simulink model "twoDofSmc"  (R2023b)
settings: Solver=VariableStepAuto  StartTime=0.0  StopTime=10.0  RelTol=1e-3
settings Model: Creator=Egraweb  LastModifiedBy=Egraweb
settings DebuggingCC: UnderSpecifiedDimensionMsg=warning

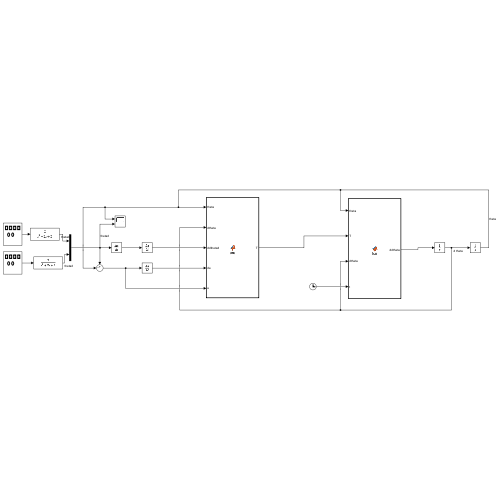
[thumbnail: Simulink's stored preview of the top-level diagram]
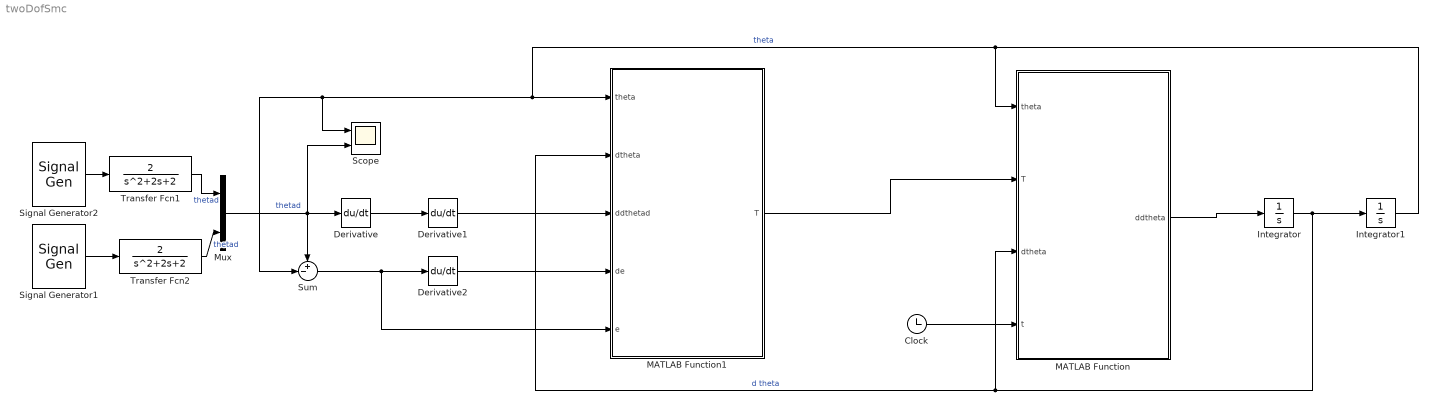
== system twoDofSmc ==
  Clock : Clock
  Derivative : Derivative
  Derivative1 : Derivative
  Derivative2 : Derivative
  Integrator : Integrator  InitialCondition=randn
  Integrator1 : Integrator  InitialCondition=randn
  MATLAB Function : MATLAB Function  TreatAsAtomicUnit=on
  MATLAB Function1 : MATLAB Function  TreatAsAtomicUnit=on
  Mux : Mux  Inputs=2
  Scope : Scope  NumInputPorts=2
  Signal Generator1 : SignalGenerator  WaveForm=square  Amplitude=2  Frequency=pi  Units=rad/sec
  Signal Generator2 : SignalGenerator  WaveForm=square  Amplitude=2  Frequency=pi  Units=rad/sec
  Sum : Sum  Inputs=+-|
  Transfer Fcn1 : TransferFcn  Numerator=[2]  Denominator=[1 2 2]
  Transfer Fcn2 : TransferFcn  Numerator=[2]  Denominator=[1 2 2]
  wires:
  MATLAB Function/1(ddtheta) -> Integrator/1
  Integrator/1 -> MATLAB Function/3(dtheta), MATLAB Function1/2(dtheta), Integrator1/1  "d theta"
  Integrator1/1 -> Scope/1, Sum/2, MATLAB Function1/1(theta), MATLAB Function/1(theta)  "theta"
  MATLAB Function1/1(T) -> MATLAB Function/2(T)
  Mux/1 -> Scope/2, Derivative/1, Sum/1  "thetad"
  Derivative/1 -> Derivative1/1
  Derivative1/1 -> MATLAB Function1/3(ddthetad)
  Sum/1 -> MATLAB Function1/5(e), Derivative2/1
  Derivative2/1 -> MATLAB Function1/4(de)
  Transfer Fcn2/1 -> Mux/2  "thetad"
  Transfer Fcn1/1 -> Mux/1  "thetad"
  Signal Generator2/1 -> Transfer Fcn1/1
  Signal Generator1/1 -> Transfer Fcn2/1
  Clock/1 -> MATLAB Function/4(t)

== matlab function twoDofSmc/MATLAB Function1 ==
  data: theta input; T output; dtheta input; ddthetad input; de input; e input
function T = smc(theta , dtheta , ddthetad , de , e)

m1 = 1; m2 = 2;
L1 = 1; L2 = 1.2;
Lc1 = 0.5; Lc2 = 0.6;
I1 = 0.15; I2 = 0.3;
g = 9.8;
D=10;

T = [0; 0];

eps = 10 * eye(2);
c = 10 * eye(2);

theta1 = theta(1); theta2 = theta(2);
dtheta1 = dtheta(1); dtheta2 = dtheta(2);


H11 = m1 * Lc1 ^2 + m2 * (Lc2^2 + L1^2 + 2 * L1 * Lc2 * cos(theta2) + I1 + I2 );
H12 = m2 * (Lc2 ^ 2 + m2 * L1 * Lc2 * cos(theta2) + I2);
H21 = H12;
H22 = m2 * Lc2 ^ 2 + I2;

c11 = -m2 * L1 * Lc2 * sin(theta2) * dtheta1;
c12 = -m2 * L1 * Lc2 * sin(theta2) * (dtheta1 + dtheta2);
c21 = m2 * L1 * Lc2 * sin (theta2) * dtheta1;

G1 = m1 * g * Lc1 * cos(theta1) + m2 * g * (L1 * cos(theta1) + Lc2* cos (theta1));
G2 = m2 * g * L2 * cos(theta1 + theta2);

H=[H11, H12;...
   H21, H22 ];
C=[c11 c12;...
    c21 0];
G=[G1; G2];

s = de + c*e;

T = H * (ddthetad + c * de + (eps + D) * sign(s) ) + C * dtheta + G;

== matlab function twoDofSmc/MATLAB Function ==
  data: theta input; T input; ddtheta output; dtheta input; t input
function ddtheta = fcn(theta ,T , dtheta ,t)

ddtheta = [0;0];
d = 10 * sin(pi*t);
m1 = 1; m2 = 2;
L1 = 1; L2 = 1.2;
Lc1 = 0.5; Lc2 = 0.6;
I1 = 0.15; I2 = 0.3;
g = 9.8;

theta1 = theta(1); theta2 = theta(2);
dtheta1 = dtheta(1); dtheta2 = dtheta(2);


H11 = m1 * Lc1 ^2 + m2 * (Lc2^2 + L1^2 + 2 * L1 * Lc2 * cos(theta2) + I1 + I2 );
H12 = m2 * (Lc2 ^ 2 + m2 * L1 * Lc2 * cos(theta2) + I2);
H21 = H12;
H22 = m2 * Lc2 ^ 2 + I2;

c11 = -m2 * L1 * Lc2 * sin(theta2) * dtheta1;
c12 = -m2 * L1 * Lc2 * sin(theta2) * (dtheta1 + dtheta2);
c21 = m2 * L1 * Lc2 * sin (theta2) * dtheta1;

G1 = m1 * g * Lc1 * cos(theta1) + m2 * g * (L1 * cos(theta1) + Lc2* cos (theta1));
G2 = m2 * g * L2 * cos(theta1 + theta2);

H=[H11, H12;...
   H21, H22 ];
C=[c11 c12;...
    c21 0];
G=[G1; G2];

ddtheta = H\ ( T - C * dtheta - G) + d;
